simulink subsystem "buoyancy_force"  (R2020a)
settings: Solver=VariableStepAuto  StartTime=0.0  StopTime=10.0  RelTol=1e-3
settings Model: Creator=Philip  LastModifiedBy=Philip

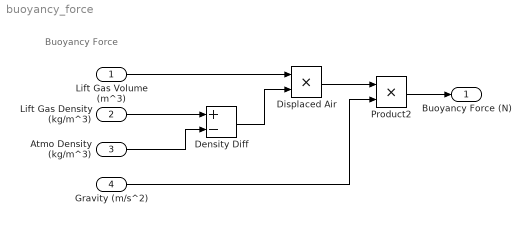
== system buoyancy_force ==
  note: Buoyancy Force
  Lift Gas Volume (m^3) : Inport
  Lift Gas Density (kg/m^3) : Inport  Port=2
  Atmo Density (kg/m^3) : Inport  Port=3
  Gravity (m/s^2) : Inport  Port=4
  Density Diff : Sum  Inputs=+-
  Displaced Air : Product
  Product2 : Product
  Buoyancy Force (N) : Outport
  wires:
  Lift Gas Volume (m^3)/1 -> Displaced Air/1
  Lift Gas Density (kg/m^3)/1 -> Density Diff/1
  Atmo Density (kg/m^3)/1 -> Density Diff/2
  Density Diff/1 -> Displaced Air/2
  Displaced Air/1 -> Product2/1
  Gravity (m/s^2)/1 -> Product2/2
  Product2/1 -> Buoyancy Force (N)/1
